simulink model "buck_converter_closed_loop_ev_accessories"  (R2019a)
settings: Solver=ode23tb  StartTime=0.0  StopTime=0.15  MaxStep=1e-7  RelTol=1e-7
values from neighbouring files (symbols this model uses):
  C = 100e-6    (= 0.0001)    [parameters_closed_loop_with_various_load.m]
  fsw = 100e3    (= 100000)    [parameters_closed_loop_with_various_load.m]
  Gco = sqrt((1+(wc/wp)^2)/(1+(wc/wz)^2))/Tuo    [parameters_closed_loop_with_various_load.m]
  H = 1    [parameters_closed_loop_with_various_load.m]
  L = 4e-3    (= 0.004)    [parameters_closed_loop_with_various_load.m]
  R_noload = V/I    (= 120000)    [parameters_closed_loop_with_various_load.m]
  Resr = 10e-3    (= 0.01)    [parameters_closed_loop_with_various_load.m]
  RL = 100e-3    (= 0.1)    [parameters_closed_loop_with_various_load.m]
  V = 12    [parameters_closed_loop_with_various_load.m]
  Vg = 72    [parameters_closed_loop_with_various_load.m]
  Vm = 1    [parameters_closed_loop_with_various_load.m]
  wL = 0    [parameters_closed_loop_with_various_load.m]
  wp = 2*pi*fp    [parameters_closed_loop_with_various_load.m]
  wz = 2*pi*fz    [parameters_closed_loop_with_various_load.m]
libraries: powerlib x20, simulink x13, powerlib_meascontrol x1, simulink_extras x1
settings Model: Creator=Görkem  LastModifiedBy=gsahi
settings SolverCC: ZeroCrossAlgorithm=Adaptive
settings DebuggingCC: IgnoredZcDiagnostic=none

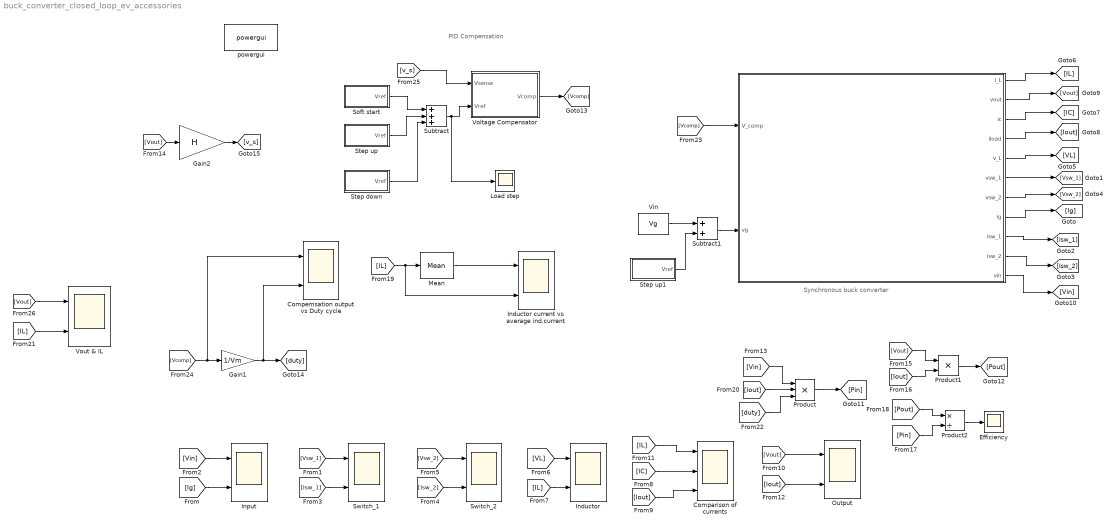
== system buck_converter_closed_loop_ev_accessories ==
  note: PID Compensation
  note: Synchronous buck converter
  "   " : Subsystem
  Comparison of currents : Scope  NumInputPorts=3
  Compemsation output vs Duty cycle : Scope  NumInputPorts=2
  Efficiency : Scope
  Gain1 : Gain  Gain=1/Vm
  Gain2 : Gain  Gain=H
  Inductor : Scope  NumInputPorts=2
  Inductor current vs average ind.current : Scope  NumInputPorts=2
  Input : Scope  NumInputPorts=2
  Load step : Scope
  Mean : powerlib_meascontrol/Measurements/Mean  Freq=fsw  Vinit=0  Ts=0
      settings: SourceProductName=Simscape Electrical
  "Output " : Scope  NumInputPorts=2
  Product : Product  Inputs=3
  Product1 : Product
  Product2 : Product  Inputs=*/
  "Soft start " : Subsystem
  Step down : Subsystem
  Step up : Subsystem
  Step up1 : Subsystem
  Subtract : Sum  Inputs=+++
  Subtract1 : Sum
  Switch_1 : Scope  NumInputPorts=2
  Switch_2 : Scope  NumInputPorts=2
  Vin : Constant  Value=Vg
  Voltage Compensator : Subsystem
  Vout & IL : Scope  NumInputPorts=2
  powergui : powerlib/powergui  Priority=1  SimulationMode=Continuous  SampleTime=5e-6  frequency=60  Iterations=50  frequencyindice=0  Pbase=100e6  ErrMax=1e-4  UnitsV=kV  UnitsW=MW  buscounter=0  FunctionMessages=off  echomessages=off  EnableUseOfTLC=off  CurrentSourceSwitches=off  DisableSnubberDevices=off  DisableRonSwitches=off  DisableVfSwitches=off  DisplayEquations=off  AutomaticDiscreteSolvers=off  SolverType=Tustin/Backward Euler (TBE)  Interpol=off  ExternalGateDelay=off  methode=off  Ts=100  x0status=blocks  SPID=on  SwTol=0  HookPort=off  NonlinearTolerance=0  nMaxIteration=15  ContinueOnMaxIteration=off  RestoreLinks=warning  ResistiveCurrentMeasurement=off  Frange=[0:2:500]  Ylog=off  Xlog=on  ShowGrid=off  save=off  variable=ZData  structure=0  ZoomFFT=off  StartTime=0.0  cycles=1  DisplayStyle=1  fundamental=60  FreqAxis=off  MaxFrequency=1000  frequencyindicesteady=1  RmsSteady=1  display=off
      settings: SourceProductName=Simscape Electrical
  wires:
  [Vsw_1] -> Switch_1/1
  [Isw_1] -> Switch_1/2
  [Vsw_2] -> Switch_2/1
  [Isw_2] -> Switch_2/2
  [VL] -> Inductor/1
  [IL] -> Inductor/2
  [IL] -> Comparison of currents/1
  [IC] -> Comparison of currents/2
  [Iout] -> Comparison of currents/3
  [Vout] -> "Output "/1
  [Iout] -> "Output "/2
  [Vin] -> Input/1
  [Ig] -> Input/2
  [Vin] -> Product/1
  [Iout] -> Product/2
  [Vout] -> Product1/1
  [Iout] -> Product1/2
  Product1/1 -> [Pout]
  Product/1 -> [Pin]
  [Pout] -> Product2/1
  [Pin] -> Product2/2
  Product2/1 -> Efficiency/1
  [duty] -> Product/3
  "   "/4(iload) -> [Iout]
  "   "/3(ic) -> [IC]
  "   "/2(vout) -> [Vout]
  "   "/1(i_L) -> [IL]
  "   "/5(v_L) -> [VL]
  "   "/6(vsw_1) -> [Vsw_1]
  "   "/7(vsw_2) -> [Vsw_2]
  "   "/8(ig) -> [Ig]
  "   "/9(isw_1) -> [Isw_1]
  "   "/10(isw_2) -> [Isw_2]
  "   "/11(vin) -> [Vin]
  [IL] -> Inductor current vs average ind.current/2, Mean/1
  Mean/1 -> Inductor current vs average ind.current/1
  [Vcomp] -> "   "/1(V_comp)
  [Vcomp] -> Compemsation output vs Duty cycle/1, Gain1/1
  Gain1/1 -> Compemsation output vs Duty cycle/2, [duty]
  [v_s] -> Voltage Compensator/1(Vsense)
  Voltage Compensator/1(Vcomp) -> [Vcomp]
  [Vout] -> Gain2/1
  Gain2/1 -> [v_s]
  [Vout] -> Vout & IL/1
  [IL] -> Vout & IL/2
  "Soft start "/1(Vref) -> Subtract/1
  Step up/1(Vref) -> Subtract/2
  Subtract/1 -> Voltage Compensator/2(Vref), Load step/1
  Step down/1(Vref) -> Subtract/3
  Vin/1 -> Subtract1/1
  Step up1/1(Vref) -> Subtract1/2
  Subtract1/1 -> "   "/2(vg)

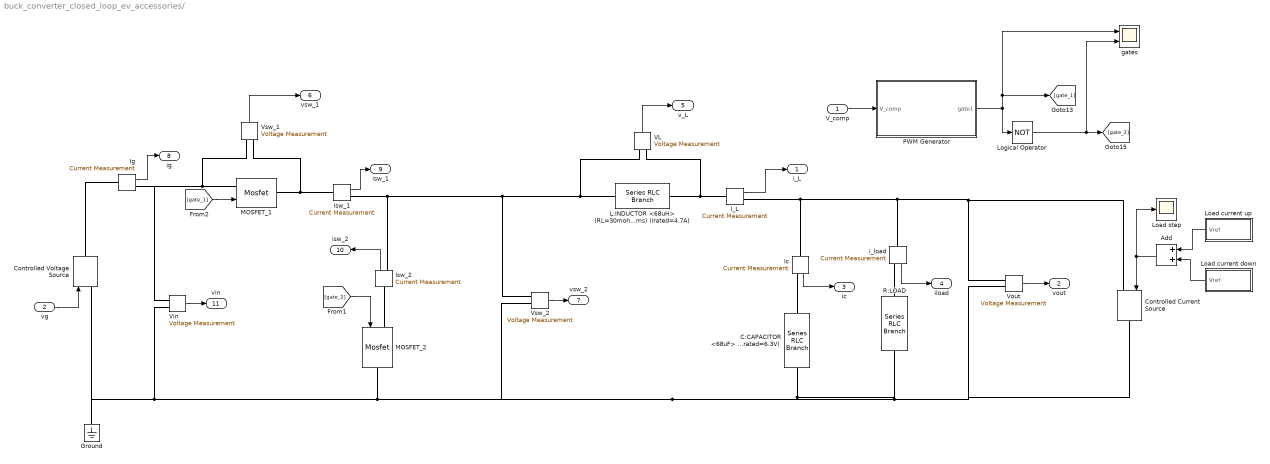
== system buck_converter_closed_loop_ev_accessories/    ==
  V_comp : Inport
  vg : Inport  Port=2
  Add : Sum
  C:CAPACITOR <68uF> (Resr=9mohms) (Vrated=6.3V) : powerlib/Elements/Series RLC Branch  LConnTagsString=__new0  RConnTagsString=__new0  BranchType=RC  Resistance=Resr  Inductance=1e-3  SetiL0=off  InitialCurrent=0  Capacitance=C  Setx0=off  InitialVoltage=0  Measurements=None
      settings: SourceProductName=Simscape Electrical
  Controlled Current Source : powerlib/Electrical Sources/Controlled Current Source  Initialize=on  Source_Type=AC  Amplitude=0  Phase=0  Frequency=0  Measurements=None
      settings: SourceProductName=Simscape Electrical
  Controlled Voltage Source : powerlib/Electrical Sources/Controlled Voltage Source  Initialize=on  Source_Type=DC  Amplitude=0  Phase=0  Frequency=0  Measurements=None
      settings: SourceProductName=Simscape Electrical
  Ground : powerlib/Elements/Ground  LConnTagsString=a
      settings: SourceProductName=Simscape Electrical
  I_L : powerlib/Measurements/Current Measurement  PhasorSimulation=off  OutputType=Complex  PSBequivalent=0
      settings: SourceProductName=Simscape Electrical
  Ic : powerlib/Measurements/Current Measurement  PhasorSimulation=off  OutputType=Complex  PSBequivalent=0
      settings: SourceProductName=Simscape Electrical
  Ig : powerlib/Measurements/Current Measurement  PhasorSimulation=off  OutputType=Complex  PSBequivalent=0
      settings: SourceProductName=Simscape Electrical
  Isw_1 : powerlib/Measurements/Current Measurement  PhasorSimulation=off  OutputType=Complex  PSBequivalent=0
      settings: SourceProductName=Simscape Electrical
  Isw_2 : powerlib/Measurements/Current Measurement  PhasorSimulation=off  OutputType=Complex  PSBequivalent=0
      settings: SourceProductName=Simscape Electrical
  "L:INDUCTOR <68uH> (RL=30mohms) (Irated=4.7A) " : powerlib/Elements/Series RLC Branch  LConnTagsString=__new0  RConnTagsString=__new0  BranchType=RL  Resistance=RL  Inductance=L  SetiL0=off  InitialCurrent=0  Capacitance=1e-6  Setx0=off  InitialVoltage=0  Measurements=None
      settings: SourceProductName=Simscape Electrical
  Load current down : Subsystem
  Load current up : Subsystem
  Load step : Scope
  Logical Operator : Logic  Operator=NOT  AllPortsSameDT=off  OutDataTypeStr=boolean
  "MOSFET_1 " : powerlib/Power Electronics/Mosfet  Ron=Rdson  Lon=0  Rd=0  Vfd=Vf  IC=0  Rs=1e5  Cs=inf  Measurements=off
      settings: SourceProductName=Simscape Electrical
  "MOSFET_2 " : powerlib/Power Electronics/Mosfet  Ron=Rdson  Lon=0  Rd=0  Vfd=Vf  IC=0  Rs=1e5  Cs=inf  Measurements=off
      settings: SourceProductName=Simscape Electrical
  PWM Generator : Subsystem
  "R:LOAD " : powerlib/Elements/Series RLC Branch  LConnTagsString=__new0  RConnTagsString=__new0  BranchType=R  Resistance=R_noload  Inductance=1e-3  SetiL0=off  InitialCurrent=0  Capacitance=47e-6  Setx0=off  InitialVoltage=0  Measurements=None
      settings: SourceProductName=Simscape Electrical
  VL : powerlib/Measurements/Voltage Measurement  PhasorSimulation=off  OutputType=Complex  PSBequivalent=0
      settings: SourceProductName=Simscape Electrical
  Vin : powerlib/Measurements/Voltage Measurement  PhasorSimulation=off  OutputType=Complex  PSBequivalent=0
      settings: SourceProductName=Simscape Electrical
  Vout : powerlib/Measurements/Voltage Measurement  PhasorSimulation=off  OutputType=Complex  PSBequivalent=0
      settings: SourceProductName=Simscape Electrical
  Vsw_1 : powerlib/Measurements/Voltage Measurement  PhasorSimulation=off  OutputType=Complex  PSBequivalent=0
      settings: SourceProductName=Simscape Electrical
  Vsw_2 : powerlib/Measurements/Voltage Measurement  PhasorSimulation=off  OutputType=Complex  PSBequivalent=0
      settings: SourceProductName=Simscape Electrical
  "gates " : Scope  NumInputPorts=2
  i_load : powerlib/Measurements/Current Measurement  PhasorSimulation=off  OutputType=Complex  PSBequivalent=0
      settings: SourceProductName=Simscape Electrical
  i_L : Outport
  vout : Outport  Port=2
  ic : Outport  Port=3
  iload : Outport  Port=4
  v_L : Outport  Port=5
  vsw_1 : Outport  Port=6
  vsw_2 : Outport  Port=7
  ig : Outport  Port=8
  isw_1 : Outport  Port=9
  isw_2 : Outport  Port=10
  vin : Outport  Port=11
  wires:
  V_comp/1 -> PWM Generator/1("V_comp ")
  [gate_2] -> "MOSFET_2 "/1
  i_load/1 -> iload/1
  Vout/1 -> vout/1
  I_L/1 -> i_L/1
  Ic/1 -> ic/1
  Vsw_2/1 -> vsw_2/1
  [gate_1] -> "MOSFET_1 "/1
  Ig/1 -> ig/1
  Isw_1/1 -> isw_1/1
  VL/1 -> v_L/1
  Isw_2/1 -> isw_2/1
  Vin/1 -> vin/1
  Vsw_1/1 -> vsw_1/1
  vg/1 -> Controlled Voltage Source/1
  PWM Generator/1(gate1) -> Logical Operator/1, "gates "/1, [gate_1]
  Logical Operator/1 -> "gates "/2, [gate_2]
  Add/1 -> Load step/1, Controlled Current Source/1
  Load current up/1(Vref) -> Add/1
  Load current down/1(Vref) -> Add/2
  connections:
  "MOSFET_1 "/LConn1 -- Vin/LConn1 -- Ig/RConn1 -- Vsw_1/LConn1
  Isw_1/RConn1 -- Isw_2/RConn1 -- Vsw_2/LConn1 -- "L:INDUCTOR <68uH> (RL=30mohms) (Irated=4.7A) "/LConn1 -- VL/LConn1
  I_L/RConn1 -- i_load/LConn1 -- Controlled Current Source/LConn1 -- Vout/LConn1 -- Ic/LConn1
  Controlled Voltage Source/RConn1 -- Ig/LConn1
  I_L/LConn1 -- VL/LConn2 -- "L:INDUCTOR <68uH> (RL=30mohms) (Irated=4.7A) "/RConn1
  Vsw_1/LConn2 -- Isw_1/LConn1 -- "MOSFET_1 "/RConn1
  "MOSFET_2 "/LConn1 -- Isw_2/LConn1
  Ic/RConn1 -- C:CAPACITOR <68uF> (Resr=9mohms) (Vrated=6.3V)/LConn1
  i_load/RConn1 -- "R:LOAD "/LConn1
  Controlled Voltage Source/LConn1 -- Ground/LConn1 -- Vin/LConn2 -- "R:LOAD "/RConn1 -- Controlled Current Source/RConn1 -- Vout/LConn2 -- C:CAPACITOR <68uF> (Resr=9mohms) (Vrated=6.3V)/RConn1 -- Vsw_2/LConn2 -- "MOSFET_2 "/RConn1

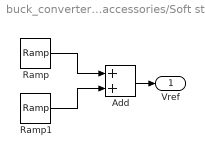
== system buck_converter_closed_loop_ev_accessories/Soft start  ==
  Add : Sum
  Ramp : simulink/Sources/Ramp  slope=(H*V)/(1000e-6)  start=0  InitialOutput=0
  Ramp1 : simulink/Sources/Ramp  slope=-(H*V)/(1000e-6)  start=1000e-6  InitialOutput=0
  Vref : Outport
  wires:
  Add/1 -> Vref/1
  Ramp/1 -> Add/1
  Ramp1/1 -> Add/2

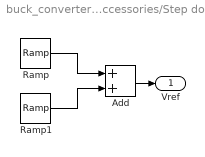
== system buck_converter_closed_loop_ev_accessories/Step down ==
  Add : Sum
  Ramp : simulink/Sources/Ramp  slope=(-1)/(1e-6)  start=0.04  InitialOutput=0
  Ramp1 : simulink/Sources/Ramp  slope=(1)/(1e-6)  start=0.04+1e-6  InitialOutput=0
  Vref : Outport
  wires:
  Add/1 -> Vref/1
  Ramp/1 -> Add/1
  Ramp1/1 -> Add/2

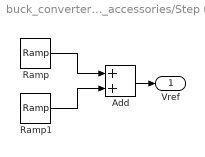
== system buck_converter_closed_loop_ev_accessories/Step up ==
  Add : Sum
  Ramp : simulink/Sources/Ramp  slope=(1)/(1e-6)  start=0.02  InitialOutput=0
  Ramp1 : simulink/Sources/Ramp  slope=-(1)/(1e-6)  start=0.02+1e-6  InitialOutput=0
  Vref : Outport
  wires:
  Add/1 -> Vref/1
  Ramp/1 -> Add/1
  Ramp1/1 -> Add/2

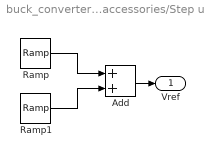
== system buck_converter_closed_loop_ev_accessories/Step up1 ==
  Add : Sum
  Ramp : simulink/Sources/Ramp  slope=(1)/(1e-6)  start=0.12  InitialOutput=0
  Ramp1 : simulink/Sources/Ramp  slope=-(1)/(1e-6)  start=0.12+1e-6  InitialOutput=0
  Vref : Outport
  wires:
  Add/1 -> Vref/1
  Ramp/1 -> Add/1
  Ramp1/1 -> Add/2

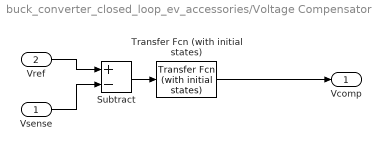
== system buck_converter_closed_loop_ev_accessories/Voltage Compensator ==
  Vsense : Inport
  Vref : Inport  Port=2
  Subtract : Sum  Inputs=+-
  Transfer Fcn (with initial states) : simulink_extras/Additional Linear/Transfer Fcn (with initial states)  N=[(Gco*wp) (Gco*wp*(wL+wz)) (Gco*wL*wz*wp)]  D=[wz (wz*wp) 0]  X0=0
  Vcomp : Outport
  wires:
  Subtract/1 -> Transfer Fcn (with initial states)/1
  Vref/1 -> Subtract/1
  Vsense/1 -> Subtract/2
  Transfer Fcn (with initial states)/1 -> Vcomp/1

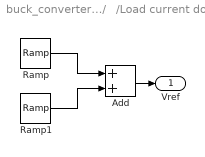
== system buck_converter_closed_loop_ev_accessories/   /Load current down ==
  Add : Sum
  Ramp : simulink/Sources/Ramp  slope=(-0.5)/(1e-6)  start=0.09  InitialOutput=0
  Ramp1 : simulink/Sources/Ramp  slope=(0.5)/(1e-6)  start=0.09+1e-6  InitialOutput=0
  Vref : Outport
  wires:
  Add/1 -> Vref/1
  Ramp/1 -> Add/1
  Ramp1/1 -> Add/2

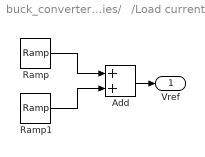
== system buck_converter_closed_loop_ev_accessories/   /Load current up ==
  Add : Sum
  Ramp : simulink/Sources/Ramp  slope=(0.5)/(1e-6)  start=0.07  InitialOutput=0
  Ramp1 : simulink/Sources/Ramp  slope=-(0.5)/(1e-6)  start=0.07+1e-6  InitialOutput=0
  Vref : Outport
  wires:
  Add/1 -> Vref/1
  Ramp/1 -> Add/1
  Ramp1/1 -> Add/2

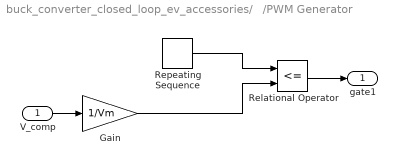
== system buck_converter_closed_loop_ev_accessories/   /PWM Generator ==
  "V_comp " : Inport
  Gain : Gain  Gain=1/Vm
  Relational Operator : RelationalOperator  Operator=<=  OutDataTypeStr=boolean  RndMeth=Simplest
  Repeating Sequence : simulink/Sources/Repeating Sequence  rep_seq_t=[0 0.5/fsw 1/fsw]  rep_seq_y=[0 Vm 0]
  gate1 : Outport
  wires:
  Repeating Sequence/1 -> Relational Operator/1
  Relational Operator/1 -> gate1/1
  "V_comp "/1 -> Gain/1
  Gain/1 -> Relational Operator/2
